simulink model "BMS_MAIN"  (R2023b)
settings: configuration reference "Configuration" (kept outside this file)
libraries: simulink x1
settings Model: DataDictionary=BMS_MAIN.sldd  Creator=Somashekar M  LastModifiedBy=Somashekar M
settings ConfigSetRef: SourceName=Configuration

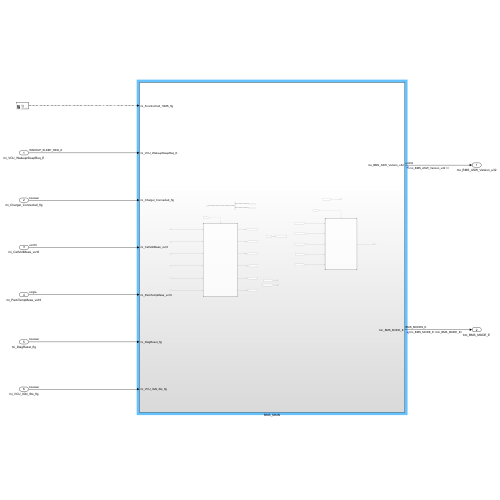
[thumbnail: Simulink's stored preview of the top-level diagram]
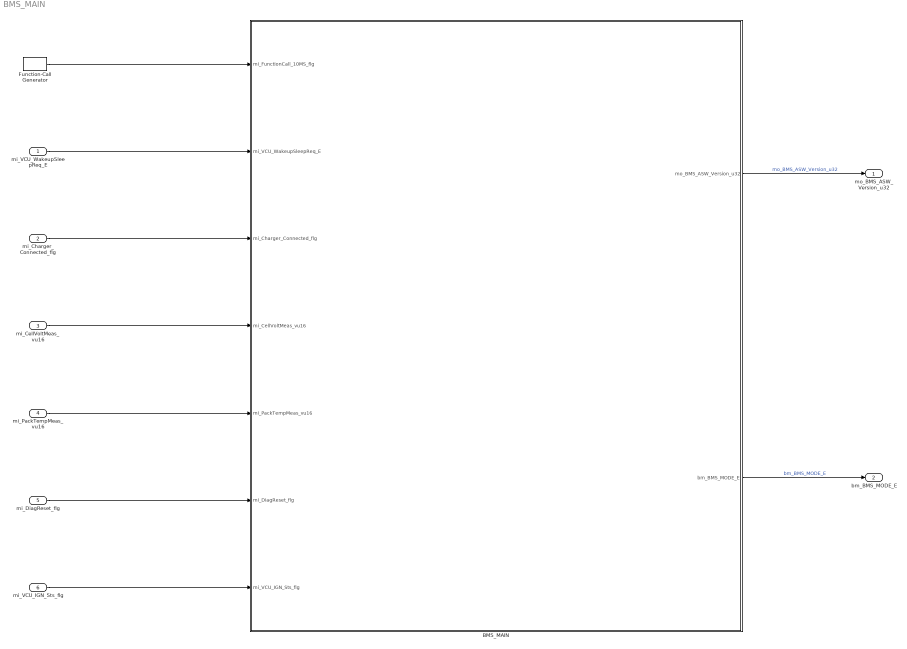
== system BMS_MAIN ==
  mi_VCU_WakeupSleepReq_E : Inport
  mi_Charger_Connected_flg : Inport  Port=2
  mi_CellVoltMeas_vu16 : Inport  Port=3
  mi_PackTempMeas_vu16 : Inport  Port=4
  mi_DiagReset_flg : Inport  Port=5
  mi_VCU_IGN_Sts_flg : Inport  Port=6
  BMS_MAIN : Subsystem
  Function-Call Generator : simulink/Ports & Subsystems/Function-Call Generator  sample_time=0.01  numberOfIterations=1  DisallowWideOutput=off
  mo_BMS_ASW_Version_u32 : Outport
  bm_BMS_MODE_E : Outport  Port=2
  wires:
  mi_Charger_Connected_flg/1 -> BMS_MAIN/3(mi_Charger_Connected_flg)
  Function-Call Generator/1 -> BMS_MAIN/1(mi_FunctionCall_10MS_flg)
  mi_VCU_IGN_Sts_flg/1 -> BMS_MAIN/7(mi_VCU_IGN_Sts_flg)
  mi_VCU_WakeupSleepReq_E/1 -> BMS_MAIN/2(mi_VCU_WakeupSleepReq_E)
  mi_DiagReset_flg/1 -> BMS_MAIN/6(mi_DiagReset_flg)
  mi_CellVoltMeas_vu16/1 -> BMS_MAIN/4(mi_CellVoltMeas_vu16)
  mi_PackTempMeas_vu16/1 -> BMS_MAIN/5(mi_PackTempMeas_vu16)
  BMS_MAIN/1(mo_BMS_ASW_Version_u32) -> mo_BMS_ASW_Version_u32/1  "mo_BMS_ASW_Version_u32"
  BMS_MAIN/2(bm_BMS_MODE_E) -> bm_BMS_MODE_E/1  "bm_BMS_MODE_E"

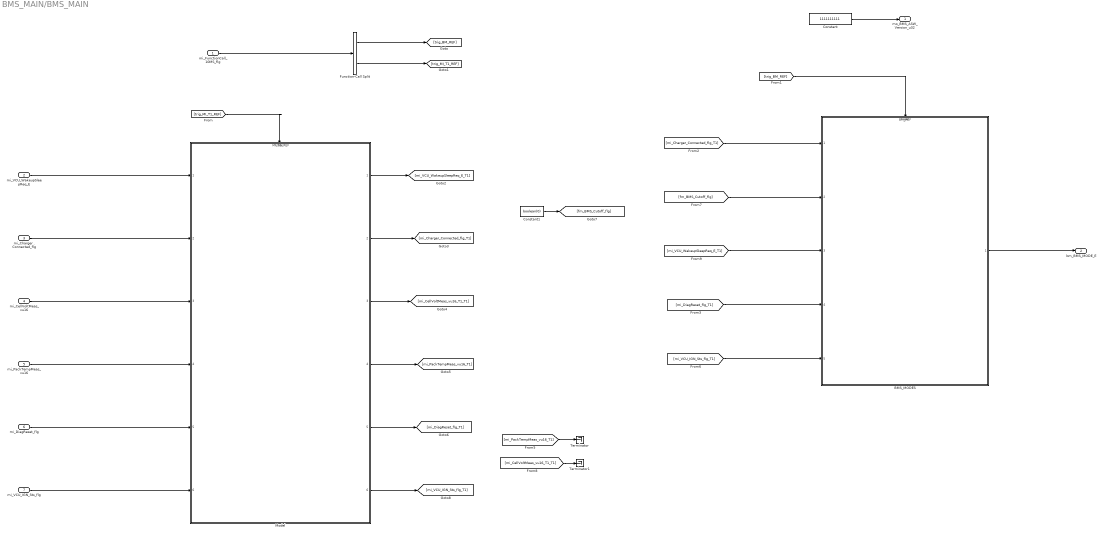
== system BMS_MAIN/BMS_MAIN ==
  mi_FunctionCall_10MS_flg : Inport
  mi_VCU_WakeupSleepReq_E : Inport  Port=2
  mi_Charger_Connected_flg : Inport  Port=3
  mi_CellVoltMeas_vu16 : Inport  Port=4
  mi_PackTempMeas_vu16 : Inport  Port=5
  mi_DiagReset_flg : Inport  Port=6
  mi_VCU_IGN_Sts_flg : Inport  Port=7
  BMS_MODES : ModelReference  ModelNameDialog=BM_REF.slx  SimulationMode=Normal  ModelReferenceVersion=1.65  TriggerPortName=function  TriggerPortTriggerType=function-call  TriggerPortStatesWhenEnabling=held
  Constant : Constant  Value=1111111111  OutDataTypeStr=uint32
  Constant1 : Constant  Value=boolean(0)
  Function-Call Split : FunctionCallSplit  IconShape=distinctive  NumOutputPorts=2  OutputPortLayout=default
  Model : ModelReference  ModelNameDialog=MI_T1_REF.slx  SimulationMode=Normal  ModelReferenceVersion=1.60  TriggerPortName=function  TriggerPortTriggerType=function-call  TriggerPortStatesWhenEnabling=held
  Terminator : Terminator
  Terminator1 : Terminator
  mo_BMS_ASW_Version_u32 : Outport
  bm_BMS_MODE_E : Outport  Port=2
  wires:
  [trig_BM_REF] -> BMS_MODES/Trigger
  [mi_Charger_Connected_flg_T1] -> BMS_MODES/1
  Function-Call Split/2 -> [trig_MI_T1_REF]
  [fm_BMS_Cutoff_flg] -> BMS_MODES/2
  [mi_VCU_WakeupSleepReq_E_T1] -> BMS_MODES/3
  mi_FunctionCall_10MS_flg/1 -> Function-Call Split/1
  Constant/1 -> mo_BMS_ASW_Version_u32/1
  Function-Call Split/1 -> [trig_BM_REF]
  [trig_MI_T1_REF] -> Model/Trigger
  mi_PackTempMeas_vu16/1 -> Model/4
  mi_CellVoltMeas_vu16/1 -> Model/3
  mi_Charger_Connected_flg/1 -> Model/2
  mi_VCU_WakeupSleepReq_E/1 -> Model/1
  Model/1 -> [mi_VCU_WakeupSleepReq_E_T1]
  Model/2 -> [mi_Charger_Connected_flg_T1]
  Model/3 -> [mi_CellVoltMeas_vu16_T1_T1]
  Model/4 -> [mi_PackTempMeas_vu16_T1]
  mi_DiagReset_flg/1 -> Model/5
  Model/5 -> [mi_DiagReset_flg_T1]
  [mi_DiagReset_flg_T1] -> BMS_MODES/4
  Constant1/1 -> [fm_BMS_Cutoff_flg]
  [mi_PackTempMeas_vu16_T1] -> Terminator/1
  [mi_CellVoltMeas_vu16_T1_T1] -> Terminator1/1
  BMS_MODES/1 -> bm_BMS_MODE_E/1
  mi_VCU_IGN_Sts_flg/1 -> Model/6
  Model/6 -> [mi_VCU_IGN_Sts_flg_T1]
  [mi_VCU_IGN_Sts_flg_T1] -> BMS_MODES/5
